simulink model "headagent"  (Simulink 6.2)
settings: Solver=ode45  StartTime=0.0  StopTime=10.0  RelTol=1e-3
settings Model: LastModifiedBy=suarezjl
settings DataIOCC: SignalLoggingName=sigsOut
settings HardwareCC: TargetUnknown=on

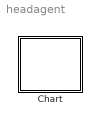
== system headagent ==
  Chart : Stateflow chart

== stateflow chart Chart ==
  state Initialize
    \\Sally\HeadTrackingDemo\HeadAgent\EyeMotionControl.Initial()
  state MainLoop
    \\Sally\HeadTrackingDemo\HeadAgent\EyeMotionControl.HeadSample()
    \\Sally\HeadTrackingDemo\HeadAgent\EyeMotionControl.DoProportionalTracking()
    \\Sally\HeadTrackingDemo\HeadAgent\EyeMotionControl.WriteMotorPositions()
    \\Sally\HeadTrackingDemo\HeadAgent\DepthEstimator.FindCartesianCoordinates()
  Initialize -> MainLoop : Always
  MainLoop -> MainLoop : Always
  (default) -> Initialize : Start
